simulink model "CA1180729"  (R2019a)
settings: Solver=VariableStepAuto  StartTime=0.0  StopTime=10.0  RelTol=1e-3
InitFcn:
  | Kpot=0.318
  | K1=100
  | a=100
  | am=1.71
  | Km=2.083
  | Kg=0.1
model workspace (MAT data in the model file):
  Kpot = Simulink.Parameter
  Kpot.DataType = 'auto'
  Kpot.Dimensions = [0 0]
values from neighbouring files (symbols this model uses):
  K = -74    [proj.m]
settings Model: Creator=totim  LastModifiedBy=totim

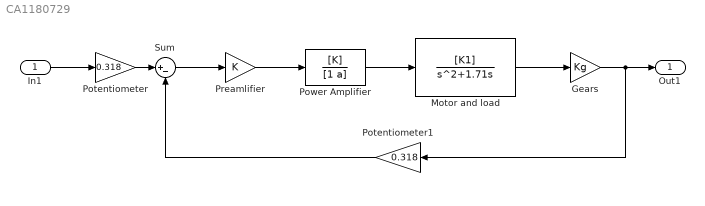
== system CA1180729 ==
  In1 : Inport
  "Gears " : Gain  Gain=Kg
  Motor and load : TransferFcn  Numerator=[K1]  Denominator=[1 1.71 0]
  Potentiometer : Gain  Gain=0.318
  Potentiometer1 : Gain  Gain=0.318
  Power Amplifier : TransferFcn  Numerator=[K]  Denominator=[1 a]
  Preamlifier : Gain  Gain=K
  Sum : Sum  Inputs=|+-
  Out1 : Outport
  wires:
  In1/1 -> Potentiometer/1
  Potentiometer/1 -> Sum/1
  Potentiometer1/1 -> Sum/2
  Sum/1 -> Preamlifier/1
  Preamlifier/1 -> Power Amplifier/1
  Power Amplifier/1 -> Motor and load/1
  "Gears "/1 -> Potentiometer1/1, Out1/1
  Motor and load/1 -> "Gears "/1
